simulink model "CarE_Model"  (R2019b)
settings: Solver=VariableStepAuto  StartTime=0.0  StopTime=inf  RelTol=1e-3
(part 2 of 5)

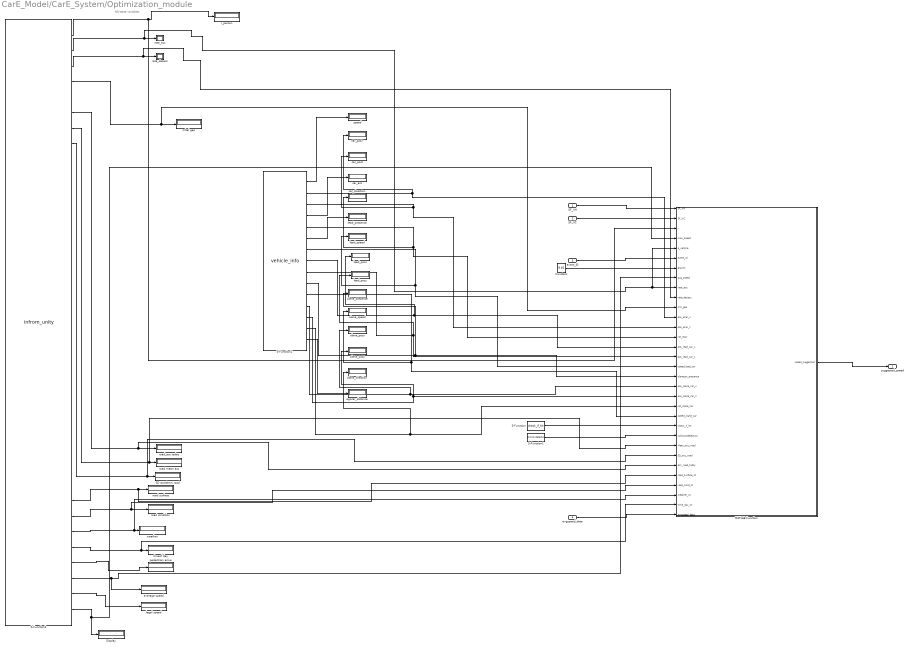
== system CarE_Model/CarE_System/Optimization_module ==
  note: NO-state variables
  SF_VH : Inport
  SF_VC : Inport  Port=2
  event_ID : Inport  Port=3
  avgspeed_data : Inport  Port=4
  Constant : Constant  Value=9.81
  Display : Display
  MATLAB Function : MATLAB Function  TreatAsAtomicUnit=on
  S-Function : S-Function  FunctionName=check_if_hit  SFunctionDeploymentMode=off  EnableBusSupport=off
  S-Function1 : S-Function  FunctionName=collisiondetection  SFunctionDeploymentMode=off  EnableBusSupport=off
  S-Function2 : S-Function  FunctionName=vehicle_info  SFunctionDeploymentMode=off  EnableBusSupport=off
  S-Function3 : S-Function  FunctionName=infrom_unity  SFunctionDeploymentMode=off  EnableBusSupport=off
  SD accidenrs road : Display
  average speed : Display
  car_acc : Display
  car_direction : Display
  car_posx : Display
  car_posz : Display
  crital gap : Display
  egocar_distance : Display
  lead_posx : Display
  lead_posz : Display
  lead_presence : Display
  lead_speed : Display
      settings: Decimation=5
  legal speed : Display
  olane_direction : Display
  olane_posx : Display
  olane_posz : Display
  olane_presence : Display
  olane_speed : Display
      settings: Decimation=5
  pedestrian acive : Display
  r_person : Display
  rate_acc : Display
  rate_desacc : Display
  road condition : Display
  road mean acc : Display
  road surface : Display
  road_acc today : Display
  speed : Display
      settings: Decimation=5
  timeof day : Display
  weather : Display
  suggested_speed : Outport
  wires:
  MATLAB Function/1(speed_suggestion) -> suggested_speed/1
  S-Function3/1 -> MATLAB Function/3(r), r_person/1
  SF_VC/1 -> MATLAB Function/2(SF_VC)
  SF_VH/1 -> MATLAB Function/1(SF_VH)
  S-Function3/38 -> MATLAB Function/4(max_speed), Display/1
  event_ID/1 -> MATLAB Function/6(event_id)
  Constant/1 -> MATLAB Function/7(gravity)
  S-Function3/36 -> average speed/1, MATLAB Function/8(avg_speed)
  S-Function3/2 -> MATLAB Function/5(a_vehicle), MATLAB Function/9(rate_acc), rate_acc/1
  S-Function3/3 -> MATLAB Function/10(rate_desacc), rate_desacc/1
  S-Function3/4 -> MATLAB Function/11(crit_gap), crital gap/1
  S-Function/1 -> MATLAB Function/23(check_if_hit)
  S-Function1/1 -> MATLAB Function/24(collisiondetection)
  S-Function3/7 -> MATLAB Function/25(Mean_acc_road), road mean acc/1
  S-Function3/8 -> MATLAB Function/26(SD_acc_road), SD accidenrs road/1
  S-Function3/6 -> MATLAB Function/27(acc_road_today), road_acc today/1
  S-Function3/31 -> MATLAB Function/28(road_surface_st), road surface/1
  S-Function3/32 -> MATLAB Function/29(road_cond_st), road condition/1
  S-Function3/33 -> MATLAB Function/30(weather_st), weather/1
  S-Function3/34 -> MATLAB Function/31(time_day_st), timeof day/1
  avgspeed_data/1 -> MATLAB Function/32(avgspeed_data)
  S-Function2/6 -> lead_presence/1
  S-Function2/11 -> MATLAB Function/22(speed_olane_car), olane_speed/1
  S-Function2/5 -> MATLAB Function/14(rot_ecar), car_direction/1
  S-Function2/8 -> MATLAB Function/15(pos_lead_car_x), lead_posx/1
  S-Function2/9 -> MATLAB Function/16(pos_lead_car_z), lead_posz/1
  S-Function2/12 -> MATLAB Function/19(pos_olane_car_x), olane_posx/1
  S-Function2/13 -> MATLAB Function/20(pos_olane_car_z), olane_posz/1
  S-Function2/15 -> egocar_distance/1
  S-Function2/7 -> MATLAB Function/17(speed_lead_car), lead_speed/1
  S-Function2/14 -> MATLAB Function/21(rot_olane_car), olane_direction/1
  S-Function2/2 -> MATLAB Function/12(pos_ecar_x), car_posx/1
  S-Function2/10 -> MATLAB Function/18(olanecar_presence), olane_presence/1
  S-Function2/3 -> MATLAB Function/13(pos_ecar_z), car_posz/1
  S-Function2/1 -> speed/1
  S-Function3/37 -> legal speed/1
  S-Function3/35 -> pedestrian acive/1
  S-Function2/4 -> car_acc/1

== system CarE_Model/CarE_System/Output Module ==
  mood : Inport
  anger_val : Inport  Port=2
  disgust_val : Inport  Port=3
  fear_val : Inport  Port=4
  happiness_val : Inport  Port=5
  neutral_val : Inport  Port=6
  sadness_val : Inport  Port=7
  surprise_val : Inport  Port=8
  stress_val : Inport  Port=9
  Body_mapping : Subsystem
  S-Function1 : S-Function  FunctionName=map_to_unity  SFunctionDeploymentMode=off  EnableBusSupport=off
  wires:
  mood/1 -> S-Function1/1
  anger_val/1 -> Body_mapping/1(anger), S-Function1/2
  disgust_val/1 -> Body_mapping/2(disgust), S-Function1/3
  fear_val/1 -> Body_mapping/3(fear), S-Function1/4
  happiness_val/1 -> Body_mapping/4(happiness), S-Function1/5
  neutral_val/1 -> Body_mapping/5(neutral), S-Function1/6
  sadness_val/1 -> Body_mapping/6(sadness), S-Function1/7
  surprise_val/1 -> Body_mapping/7(surprise), S-Function1/8
  stress_val/1 -> Body_mapping/8(stress), S-Function1/9

== system CarE_Model/CarE_System/Personality_module ==
  egocar_speed : Inport
  egocar_max_speed : Inport  Port=2
  r_personality : Inport  Port=3
  MATLAB Function : MATLAB Function  TreatAsAtomicUnit=on
  MATLAB Function1 : MATLAB Function  TreatAsAtomicUnit=on
  Utility : Outport
  wires:
  egocar_max_speed/1 -> MATLAB Function/2(max_speed)
  egocar_speed/1 -> MATLAB Function/1(speed)
  r_personality/1 -> MATLAB Function1/2(r)
  MATLAB Function/2(max_x) -> MATLAB Function1/3(max_x)
  MATLAB Function/1(x) -> MATLAB Function1/1(x)
  MATLAB Function1/1(U) -> Utility/1

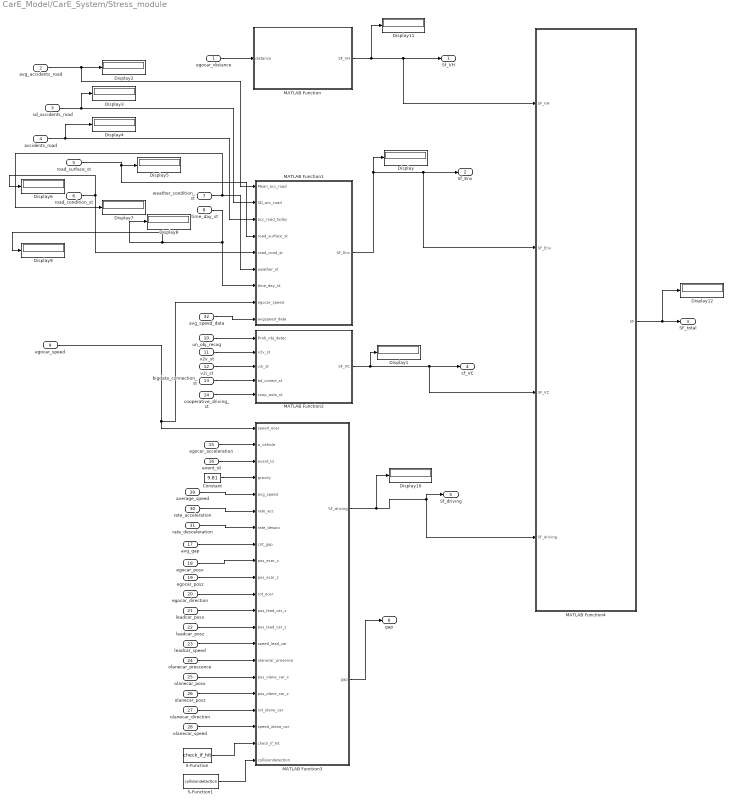
== system CarE_Model/CarE_System/Stress_module ==
  egocar_distance : Inport
  avg_accidents_road : Inport  Port=2
  sd_accidents_road : Inport  Port=3
  accidents_road : Inport  Port=4
  road_surface_st : Inport  Port=5
  road_condition_st : Inport  Port=6
  weather_condition_st : Inport  Port=7
  time_day_st : Inport  Port=8
  egocar_speed : Inport  Port=9
  un_obj_recog : Inport  Port=10
  v2v_st : Inport  Port=11
  v2i_st : Inport  Port=12
  bigdata_connection_st : Inport  Port=13
  cooperative_driving_st : Inport  Port=14
  egocar_acceleration : Inport  Port=15
  event_id : Inport  Port=16
  avg_gap : Inport  Port=17
  egocar_posx : Inport  Port=18
  egocar_posz : Inport  Port=19
  egocar_direction : Inport  Port=20
  leadcar_posx : Inport  Port=21
  leadcar_posz : Inport  Port=22
  leadcar_speed : Inport  Port=23
  olanecar_prescence : Inport  Port=24
  olanecar_posx : Inport  Port=25
  olanecar_posz : Inport  Port=26
  olanecar_direction : Inport  Port=27
  olanecar_speed : Inport  Port=28
  average_speed : Inport  Port=29
  rate_acceleration : Inport  Port=30
  rate_desceleration : Inport  Port=31
  avg_speed_data : Inport  Port=32
  Constant : Constant  Value=9.81
  Display{,1..12} (13 alike) : Display
  MATLAB Function : MATLAB Function  TreatAsAtomicUnit=on
  MATLAB Function1 : MATLAB Function  TreatAsAtomicUnit=on
  MATLAB Function2 : MATLAB Function  TreatAsAtomicUnit=on
  MATLAB Function3 : MATLAB Function  TreatAsAtomicUnit=on
  MATLAB Function4 : MATLAB Function  TreatAsAtomicUnit=on
  S-Function : S-Function  FunctionName=check_if_hit  SFunctionDeploymentMode=off  EnableBusSupport=off
  S-Function1 : S-Function  FunctionName=collisiondetection  SFunctionDeploymentMode=off  EnableBusSupport=off
  Sf_VH : Outport
  Sf_Env : Outport  Port=2
  SF_total : Outport  Port=3
  sf_VC : Outport  Port=4
  Sf_driving : Outport  Port=5
  gap : Outport  Port=6
  wires:
  MATLAB Function/1(SF_VH) -> Display11/1, MATLAB Function4/1(SF_VH), Sf_VH/1
  egocar_distance/1 -> MATLAB Function/1(distance)
  egocar_speed/1 -> MATLAB Function1/8(egocar_speed), MATLAB Function3/1(speed_ecar)
  avg_accidents_road/1 -> MATLAB Function1/1(Mean_acc_road), Display2/1
  sd_accidents_road/1 -> MATLAB Function1/2(SD_acc_road), Display3/1
  accidents_road/1 -> Display4/1, MATLAB Function1/3(acc_road_today)
  road_surface_st/1 -> MATLAB Function1/4(road_surface_st), Display5/1
  road_condition_st/1 -> Display6/1, MATLAB Function1/5(road_cond_st)
  weather_condition_st/1 -> Display7/1, MATLAB Function1/6(weather_st)
  time_day_st/1 -> Display9/1, Display8/1, MATLAB Function1/7(time_day_st)
  MATLAB Function1/1(SF_Env) -> Display/1, MATLAB Function4/2(SF_Env), Sf_Env/1
  MATLAB Function4/1(SF) -> Display12/1, SF_total/1
  MATLAB Function2/1(SF_VC) -> Display1/1, MATLAB Function4/3(SF_VC), sf_VC/1
  MATLAB Function3/1(SF_driving) -> Display10/1, Sf_driving/1, MATLAB Function4/4(SF_driving)
  cooperative_driving_st/1 -> MATLAB Function2/5(coop_auto_st)
  bigdata_connection_st/1 -> MATLAB Function2/4(bd_conect_st)
  v2i_st/1 -> MATLAB Function2/3(v2i_st)
  v2v_st/1 -> MATLAB Function2/2(v2v_st)
  un_obj_recog/1 -> MATLAB Function2/1(Prob_obj_detec)
  Constant/1 -> MATLAB Function3/4(gravity)
  event_id/1 -> MATLAB Function3/3(event_id)
  egocar_acceleration/1 -> MATLAB Function3/2(a_vehicle)
  avg_gap/1 -> MATLAB Function3/8(crit_gap)
  leadcar_speed/1 -> MATLAB Function3/14(speed_lead_car)
  leadcar_posz/1 -> MATLAB Function3/13(pos_lead_car_z)
  leadcar_posx/1 -> MATLAB Function3/12(pos_lead_car_x)
  egocar_direction/1 -> MATLAB Function3/11(rot_ecar)
  egocar_posz/1 -> MATLAB Function3/10(pos_ecar_z)
  egocar_posx/1 -> MATLAB Function3/9(pos_ecar_x)
  olanecar_speed/1 -> MATLAB Function3/19(speed_olane_car)
  olanecar_direction/1 -> MATLAB Function3/18(rot_olane_car)
  olanecar_posz/1 -> MATLAB Function3/17(pos_olane_car_z)
  olanecar_posx/1 -> MATLAB Function3/16(pos_olane_car_x)
  olanecar_prescence/1 -> MATLAB Function3/15(olanecar_presence)
  MATLAB Function3/2(gap) -> gap/1
  rate_desceleration/1 -> MATLAB Function3/7(rate_desacc)
  rate_acceleration/1 -> MATLAB Function3/6(rate_acc)
  average_speed/1 -> MATLAB Function3/5(avg_speed)
  S-Function/1 -> MATLAB Function3/20(check_if_hit)
  S-Function1/1 -> MATLAB Function3/21(collisiondetection)
  avg_speed_data/1 -> MATLAB Function1/9(avgspeed_data)

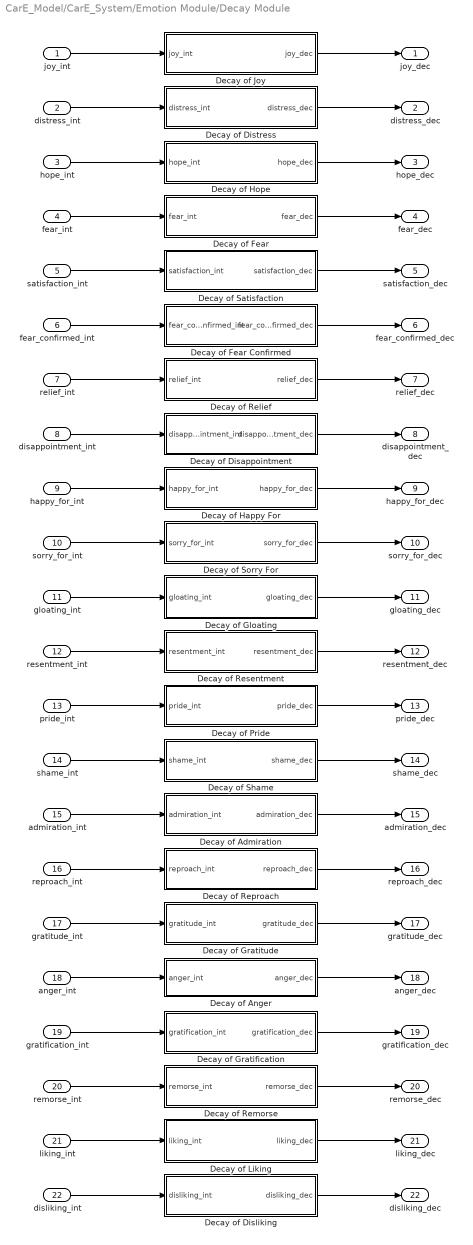
== system CarE_Model/CarE_System/Emotion Module/Decay Module ==
  joy_int : Inport
  distress_int : Inport  Port=2
  hope_int : Inport  Port=3
  fear_int : Inport  Port=4
  satisfaction_int : Inport  Port=5
  fear_confirmed_int : Inport  Port=6
  relief_int : Inport  Port=7
  disappointment_int : Inport  Port=8
  happy_for_int : Inport  Port=9
  sorry_for_int : Inport  Port=10
  gloating_int : Inport  Port=11
  resentment_int : Inport  Port=12
  pride_int : Inport  Port=13
  shame_int : Inport  Port=14
  admiration_int : Inport  Port=15
  reproach_int : Inport  Port=16
  gratitude_int : Inport  Port=17
  anger_int : Inport  Port=18
  gratification_int : Inport  Port=19
  remorse_int : Inport  Port=20
  liking_int : Inport  Port=21
  disliking_int : Inport  Port=22
  Decay of Admiration : Subsystem
  Decay of Anger : Subsystem
  Decay of Disappointment : Subsystem
  Decay of Disliking : Subsystem
  Decay of Distress : Subsystem
  Decay of Fear : Subsystem
  Decay of Fear Confirmed : Subsystem
  Decay of Gloating : Subsystem
  Decay of Gratification : Subsystem
  Decay of Gratitude : Subsystem
  Decay of Happy For : Subsystem
  Decay of Hope : Subsystem
  Decay of Joy : Subsystem
  Decay of Liking : Subsystem
  Decay of Pride : Subsystem
  Decay of Relief : Subsystem
  Decay of Remorse : Subsystem
  Decay of Reproach : Subsystem
  Decay of Resentment : Subsystem
  Decay of Satisfaction : Subsystem
  Decay of Shame : Subsystem
  Decay of Sorry For : Subsystem
  joy_dec : Outport  VectorParamsAs1DForOutWhenUnconnected=off
  "distress_dec " : Outport  Port=2  VectorParamsAs1DForOutWhenUnconnected=off
  hope_dec : Outport  Port=3  VectorParamsAs1DForOutWhenUnconnected=off
  fear_dec : Outport  Port=4  VectorParamsAs1DForOutWhenUnconnected=off
  satisfaction_dec : Outport  Port=5  VectorParamsAs1DForOutWhenUnconnected=off
  fear_confirmed_dec : Outport  Port=6  VectorParamsAs1DForOutWhenUnconnected=off
  relief_dec : Outport  Port=7  VectorParamsAs1DForOutWhenUnconnected=off
  disappointment_dec : Outport  Port=8  VectorParamsAs1DForOutWhenUnconnected=off
  happy_for_dec : Outport  Port=9  VectorParamsAs1DForOutWhenUnconnected=off
  sorry_for_dec : Outport  Port=10  VectorParamsAs1DForOutWhenUnconnected=off
  gloating_dec : Outport  Port=11  VectorParamsAs1DForOutWhenUnconnected=off
  resentment_dec : Outport  Port=12  VectorParamsAs1DForOutWhenUnconnected=off
  pride_dec : Outport  Port=13  VectorParamsAs1DForOutWhenUnconnected=off
  shame_dec : Outport  Port=14  VectorParamsAs1DForOutWhenUnconnected=off
  admiration_dec : Outport  Port=15  VectorParamsAs1DForOutWhenUnconnected=off
  reproach_dec : Outport  Port=16  VectorParamsAs1DForOutWhenUnconnected=off
  gratitude_dec : Outport  Port=17  VectorParamsAs1DForOutWhenUnconnected=off
  anger_dec : Outport  Port=18  VectorParamsAs1DForOutWhenUnconnected=off
  gratification_dec : Outport  Port=19  VectorParamsAs1DForOutWhenUnconnected=off
  remorse_dec : Outport  Port=20  VectorParamsAs1DForOutWhenUnconnected=off
  liking_dec : Outport  Port=21  VectorParamsAs1DForOutWhenUnconnected=off
  disliking_dec : Outport  Port=22  VectorParamsAs1DForOutWhenUnconnected=off
  wires:
  distress_int/1 -> Decay of Distress/1(distress_int)
  joy_int/1 -> Decay of Joy/1(joy_int)
  fear_int/1 -> Decay of Fear/1(fear_int)
  hope_int/1 -> Decay of Hope/1(hope_int)
  satisfaction_int/1 -> Decay of Satisfaction/1(satisfaction_int)
  fear_confirmed_int/1 -> Decay of Fear Confirmed/1(fear_confirmed_int)
  relief_int/1 -> Decay of Relief/1(relief_int)
  disappointment_int/1 -> Decay of Disappointment/1(disappointment_int)
  happy_for_int/1 -> Decay of Happy For/1(happy_for_int)
  sorry_for_int/1 -> Decay of Sorry For/1(sorry_for_int)
  gloating_int/1 -> Decay of Gloating/1(gloating_int)
  resentment_int/1 -> Decay of Resentment/1(resentment_int)
  pride_int/1 -> Decay of Pride/1(pride_int)
  shame_int/1 -> Decay of Shame/1(shame_int)
  admiration_int/1 -> Decay of Admiration/1(admiration_int)
  reproach_int/1 -> Decay of Reproach/1(reproach_int)
  gratitude_int/1 -> Decay of Gratitude/1(gratitude_int)
  anger_int/1 -> Decay of Anger/1(anger_int)
  gratification_int/1 -> Decay of Gratification/1(gratification_int)
  remorse_int/1 -> Decay of Remorse/1(remorse_int)
  liking_int/1 -> Decay of Liking/1(liking_int)
  disliking_int/1 -> Decay of Disliking/1(disliking_int)
  Decay of Joy/1(joy_dec) -> joy_dec/1
  Decay of Distress/1(distress_dec) -> "distress_dec "/1
  Decay of Hope/1(hope_dec) -> hope_dec/1
  Decay of Fear/1(fear_dec) -> fear_dec/1
  Decay of Satisfaction/1(satisfaction_dec) -> satisfaction_dec/1
  Decay of Fear Confirmed/1(fear_confirmed_dec) -> fear_confirmed_dec/1
  Decay of Relief/1(relief_dec) -> relief_dec/1
  Decay of Disappointment/1(disappointment_dec) -> disappointment_dec/1
  Decay of Happy For/1(happy_for_dec) -> happy_for_dec/1
  Decay of Sorry For/1(sorry_for_dec) -> sorry_for_dec/1
  Decay of Gloating/1(gloating_dec) -> gloating_dec/1
  Decay of Resentment/1(resentment_dec) -> resentment_dec/1
  Decay of Pride/1(pride_dec) -> pride_dec/1
  Decay of Shame/1(shame_dec) -> shame_dec/1
  Decay of Admiration/1(admiration_dec) -> admiration_dec/1
  Decay of Reproach/1(reproach_dec) -> reproach_dec/1
  Decay of Gratitude/1(gratitude_dec) -> gratitude_dec/1
  Decay of Anger/1(anger_dec) -> anger_dec/1
  Decay of Gratification/1(gratification_dec) -> gratification_dec/1
  Decay of Remorse/1(remorse_dec) -> remorse_dec/1
  Decay of Liking/1(liking_dec) -> liking_dec/1
  Decay of Disliking/1(disliking_dec) -> disliking_dec/1

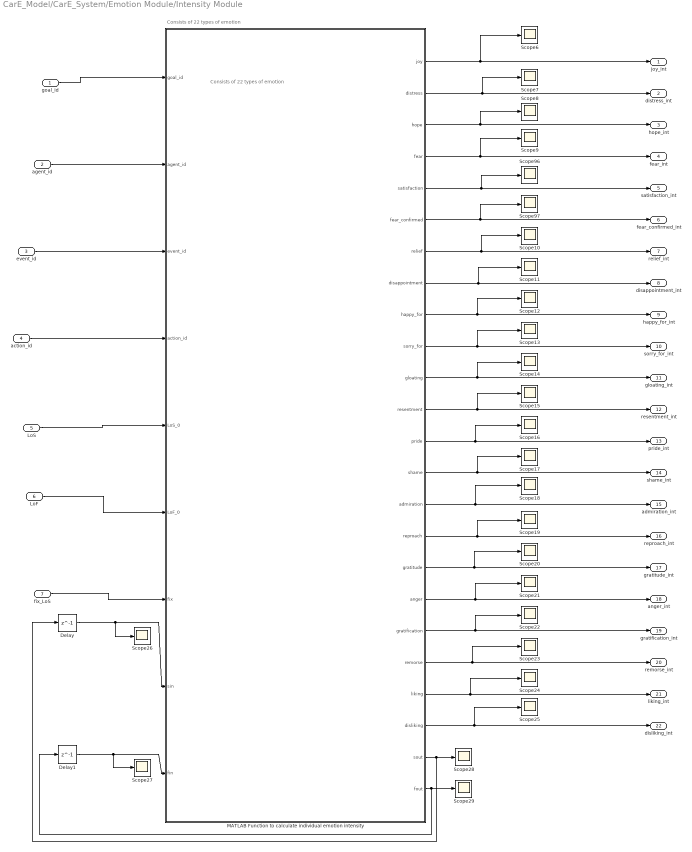
== system CarE_Model/CarE_System/Emotion Module/Intensity Module ==
  note: Consists of 22 types of emotion
  note: Consists of 22 types of emotion
  goal_id : Inport
  agent_id : Inport  Port=2
  event_id : Inport  Port=3
  action_id : Inport  Port=4
  LoS : Inport  Port=5
  LoF : Inport  Port=6
  fix_LoS : Inport  Port=7
  Delay : Delay  DelayLength=1  InitialCondition=0
  Delay1 : Delay  DelayLength=1  InitialCondition=0
  MATLAB Function to calculate individual emotion intensity : MATLAB Function  TreatAsAtomicUnit=on
  Scope{6..29,96..97} (26 alike) : Scope
  joy_int : Outport  VectorParamsAs1DForOutWhenUnconnected=off
  "distress_int " : Outport  Port=2  VectorParamsAs1DForOutWhenUnconnected=off
  hope_int : Outport  Port=3  VectorParamsAs1DForOutWhenUnconnected=off
  fear_int : Outport  Port=4  VectorParamsAs1DForOutWhenUnconnected=off
  satisfaction_int : Outport  Port=5  VectorParamsAs1DForOutWhenUnconnected=off
  fear_confirmed_int : Outport  Port=6  VectorParamsAs1DForOutWhenUnconnected=off
  relief_int : Outport  Port=7  VectorParamsAs1DForOutWhenUnconnected=off
  disappointment_int : Outport  Port=8  VectorParamsAs1DForOutWhenUnconnected=off
  happy_for_int : Outport  Port=9  VectorParamsAs1DForOutWhenUnconnected=off
  sorry_for_int : Outport  Port=10  VectorParamsAs1DForOutWhenUnconnected=off
  gloating_int : Outport  Port=11  VectorParamsAs1DForOutWhenUnconnected=off
  resentment_int : Outport  Port=12  VectorParamsAs1DForOutWhenUnconnected=off
  pride_int : Outport  Port=13  VectorParamsAs1DForOutWhenUnconnected=off
  shame_int : Outport  Port=14  VectorParamsAs1DForOutWhenUnconnected=off
  admiration_int : Outport  Port=15  VectorParamsAs1DForOutWhenUnconnected=off
  reproach_int : Outport  Port=16  VectorParamsAs1DForOutWhenUnconnected=off
  gratitude_int : Outport  Port=17  VectorParamsAs1DForOutWhenUnconnected=off
  anger_int : Outport  Port=18  VectorParamsAs1DForOutWhenUnconnected=off
  gratification_int : Outport  Port=19  VectorParamsAs1DForOutWhenUnconnected=off
  remorse_int : Outport  Port=20  VectorParamsAs1DForOutWhenUnconnected=off
  liking_int : Outport  Port=21  VectorParamsAs1DForOutWhenUnconnected=off
  disliking_int : Outport  Port=22  VectorParamsAs1DForOutWhenUnconnected=off
  wires:
  MATLAB Function to calculate individual emotion intensity/11(gloating) -> gloating_int/1, Scope14/1
  MATLAB Function to calculate individual emotion intensity/9(happy_for) -> happy_for_int/1, Scope12/1
  event_id/1 -> MATLAB Function to calculate individual emotion intensity/3(event_id)
  MATLAB Function to calculate individual emotion intensity/10(sorry_for) -> sorry_for_int/1, Scope13/1
  goal_id/1 -> MATLAB Function to calculate individual emotion intensity/1(goal_id)
  MATLAB Function to calculate individual emotion intensity/4(fear) -> fear_int/1, Scope9/1
  MATLAB Function to calculate individual emotion intensity/3(hope) -> hope_int/1, Scope8/1
  MATLAB Function to calculate individual emotion intensity/19(gratification) -> gratification_int/1, Scope22/1
  MATLAB Function to calculate individual emotion intensity/13(pride) -> pride_int/1, Scope16/1
  MATLAB Function to calculate individual emotion intensity/20(remorse) -> remorse_int/1, Scope23/1
  Delay/1 -> Scope26/1, MATLAB Function to calculate individual emotion intensity/8(sin)
  MATLAB Function to calculate individual emotion intensity/17(gratitude) -> gratitude_int/1, Scope20/1
  MATLAB Function to calculate individual emotion intensity/22(disliking) -> disliking_int/1, Scope25/1
  MATLAB Function to calculate individual emotion intensity/21(liking) -> Scope24/1, liking_int/1
  MATLAB Function to calculate individual emotion intensity/8(disappointment) -> disappointment_int/1, Scope11/1
  MATLAB Function to calculate individual emotion intensity/2(distress) -> "distress_int "/1, Scope7/1
  MATLAB Function to calculate individual emotion intensity/15(admiration) -> admiration_int/1, Scope18/1
  MATLAB Function to calculate individual emotion intensity/5(satisfaction) -> satisfaction_int/1, Scope96/1
  MATLAB Function to calculate individual emotion intensity/18(anger) -> anger_int/1, Scope21/1
  agent_id/1 -> MATLAB Function to calculate individual emotion intensity/2(agent_id)
  MATLAB Function to calculate individual emotion intensity/6(fear_confirmed) -> fear_confirmed_int/1, Scope97/1
  Delay1/1 -> Scope27/1, MATLAB Function to calculate individual emotion intensity/9(fin)
  MATLAB Function to calculate individual emotion intensity/1(joy) -> joy_int/1, Scope6/1
  MATLAB Function to calculate individual emotion intensity/16(reproach) -> reproach_int/1, Scope19/1
  action_id/1 -> MATLAB Function to calculate individual emotion intensity/4(action_id)
  MATLAB Function to calculate individual emotion intensity/12(resentment) -> resentment_int/1, Scope15/1
  MATLAB Function to calculate individual emotion intensity/14(shame) -> shame_int/1, Scope17/1
  MATLAB Function to calculate individual emotion intensity/24(fout) -> Delay1/1, Scope29/1
  MATLAB Function to calculate individual emotion intensity/7(relief) -> relief_int/1, Scope10/1
  MATLAB Function to calculate individual emotion intensity/23(sout) -> Delay/1, Scope28/1
  LoS/1 -> MATLAB Function to calculate individual emotion intensity/5(LoS_0)
  LoF/1 -> MATLAB Function to calculate individual emotion intensity/6(LoF_0)
  fix_LoS/1 -> MATLAB Function to calculate individual emotion intensity/7(fix)

== system CarE_Model/CarE_System/Output Module/Body_mapping ==
  anger : Inport
  disgust : Inport  Port=2
  fear : Inport  Port=3
  happiness : Inport  Port=4
  neutral : Inport  Port=5
  sadness : Inport  Port=6
  surprise : Inport  Port=7
  stress : Inport  Port=8
  MATLAB Function : MATLAB Function  TreatAsAtomicUnit=on
  S-Function : S-Function  FunctionName=bodymap  SFunctionDeploymentMode=off  EnableBusSupport=off
  wires:
  stress/1 -> MATLAB Function/8(stress)
  surprise/1 -> MATLAB Function/7(surprise)
  sadness/1 -> MATLAB Function/6(sadness)
  neutral/1 -> MATLAB Function/5(neutral)
  happiness/1 -> MATLAB Function/4(happiness)
  fear/1 -> MATLAB Function/3(fear)
  disgust/1 -> MATLAB Function/2(disgust)
  anger/1 -> MATLAB Function/1(anger)
  MATLAB Function/1(cabine_st) -> S-Function/1
  MATLAB Function/2(tires_st) -> S-Function/2
  MATLAB Function/3(wheels_st) -> S-Function/3
  MATLAB Function/4(motor_st) -> S-Function/4
  MATLAB Function/5(dashboard_st) -> S-Function/5
  MATLAB Function/6(door_st) -> S-Function/6
  MATLAB Function/7(body_st) -> S-Function/7
  MATLAB Function/8(windshield_st) -> S-Function/8
  MATLAB Function/9(ligths_st) -> S-Function/9
  MATLAB Function/10(comm_st) -> S-Function/10

== system CarE_Model/CarE_System/Emotion Module/Decay Module/Decay of Admiration ==
  admiration_int : Inport
  Clock : Clock
  Delay : Delay  DelayLength=1  InitialCondition=0
  MATLAB Function : MATLAB Function  TreatAsAtomicUnit=on
  admiration_dec : Outport  VectorParamsAs1DForOutWhenUnconnected=off
  wires:
  admiration_int/1 -> Delay/1, MATLAB Function/1(u)
  Clock/1 -> MATLAB Function/2(t)
  MATLAB Function/1(y) -> admiration_dec/1
  Delay/1 -> MATLAB Function/3(ulast)

== system CarE_Model/CarE_System/Emotion Module/Decay Module/Decay of Anger ==
  anger_int : Inport
  Clock : Clock
  Delay : Delay  DelayLength=1  InitialCondition=0
  MATLAB Function : MATLAB Function  TreatAsAtomicUnit=on
  anger_dec : Outport  VectorParamsAs1DForOutWhenUnconnected=off
  wires:
  Delay/1 -> MATLAB Function/3(ulast)
  Clock/1 -> MATLAB Function/2(t)
  anger_int/1 -> Delay/1, MATLAB Function/1(u)
  MATLAB Function/1(y) -> anger_dec/1

== system CarE_Model/CarE_System/Emotion Module/Decay Module/Decay of Disappointment ==
  disappointment_int : Inport
  Clock : Clock
  Delay : Delay  DelayLength=1  InitialCondition=0
  MATLAB Function : MATLAB Function  TreatAsAtomicUnit=on
  disappointment_dec : Outport  VectorParamsAs1DForOutWhenUnconnected=off
  wires:
  Delay/1 -> MATLAB Function/3(ulast)
  Clock/1 -> MATLAB Function/2(t)
  disappointment_int/1 -> Delay/1, MATLAB Function/1(u)
  MATLAB Function/1(y) -> disappointment_dec/1

== system CarE_Model/CarE_System/Emotion Module/Decay Module/Decay of Disliking ==
  disliking_int : Inport
  Clock : Clock
  Delay : Delay  DelayLength=1  InitialCondition=0
  MATLAB Function : MATLAB Function  TreatAsAtomicUnit=on
  disliking_dec : Outport  VectorParamsAs1DForOutWhenUnconnected=off
  wires:
  Delay/1 -> MATLAB Function/3(ulast)
  Clock/1 -> MATLAB Function/2(t)
  disliking_int/1 -> Delay/1, MATLAB Function/1(u)
  MATLAB Function/1(y) -> disliking_dec/1

== system CarE_Model/CarE_System/Emotion Module/Decay Module/Decay of Distress ==
  distress_int : Inport
  Clock : Clock
  Delay : Delay  DelayLength=1  InitialCondition=0
  MATLAB Function : MATLAB Function  TreatAsAtomicUnit=on
  distress_dec : Outport  VectorParamsAs1DForOutWhenUnconnected=off
  wires:
  Clock/1 -> MATLAB Function/2(t)
  MATLAB Function/1(y) -> distress_dec/1
  Delay/1 -> MATLAB Function/3(ulast)
  distress_int/1 -> Delay/1, MATLAB Function/1(u)

== system CarE_Model/CarE_System/Emotion Module/Decay Module/Decay of Fear ==
  fear_int : Inport
  Clock : Clock
  Delay : Delay  DelayLength=1  InitialCondition=0
  MATLAB Function : MATLAB Function  TreatAsAtomicUnit=on
  fear_dec : Outport  VectorParamsAs1DForOutWhenUnconnected=off
  wires:
  Delay/1 -> MATLAB Function/3(ulast)
  Clock/1 -> MATLAB Function/2(t)
  fear_int/1 -> Delay/1, MATLAB Function/1(u)
  MATLAB Function/1(y) -> fear_dec/1

== system CarE_Model/CarE_System/Emotion Module/Decay Module/Decay of Fear Confirmed ==
  fear_confirmed_int : Inport
  Clock : Clock
  Delay : Delay  DelayLength=1  InitialCondition=0
  MATLAB Function : MATLAB Function  TreatAsAtomicUnit=on
  fear_confirmed_dec : Outport  VectorParamsAs1DForOutWhenUnconnected=off
  wires:
  Delay/1 -> MATLAB Function/3(ulast)
  Clock/1 -> MATLAB Function/2(t)
  fear_confirmed_int/1 -> Delay/1, MATLAB Function/1(u)
  MATLAB Function/1(y) -> fear_confirmed_dec/1

== system CarE_Model/CarE_System/Emotion Module/Decay Module/Decay of Gloating ==
  gloating_int : Inport
  Clock : Clock
  Delay : Delay  DelayLength=1  InitialCondition=0
  MATLAB Function : MATLAB Function  TreatAsAtomicUnit=on
  gloating_dec : Outport  VectorParamsAs1DForOutWhenUnconnected=off
  wires:
  Delay/1 -> MATLAB Function/3(ulast)
  Clock/1 -> MATLAB Function/2(t)
  gloating_int/1 -> Delay/1, MATLAB Function/1(u)
  MATLAB Function/1(y) -> gloating_dec/1

== system CarE_Model/CarE_System/Emotion Module/Decay Module/Decay of Gratification ==
  gratification_int : Inport
  Clock : Clock
  Delay : Delay  DelayLength=1  InitialCondition=0
  MATLAB Function : MATLAB Function  TreatAsAtomicUnit=on
  gratification_dec : Outport  VectorParamsAs1DForOutWhenUnconnected=off
  wires:
  Delay/1 -> MATLAB Function/3(ulast)
  Clock/1 -> MATLAB Function/2(t)
  gratification_int/1 -> Delay/1, MATLAB Function/1(u)
  MATLAB Function/1(y) -> gratification_dec/1

== system CarE_Model/CarE_System/Emotion Module/Decay Module/Decay of Gratitude ==
  gratitude_int : Inport
  Clock : Clock
  Delay : Delay  DelayLength=1  InitialCondition=0
  MATLAB Function : MATLAB Function  TreatAsAtomicUnit=on
  gratitude_dec : Outport  VectorParamsAs1DForOutWhenUnconnected=off
  wires:
  Delay/1 -> MATLAB Function/3(ulast)
  Clock/1 -> MATLAB Function/2(t)
  gratitude_int/1 -> Delay/1, MATLAB Function/1(u)
  MATLAB Function/1(y) -> gratitude_dec/1

== system CarE_Model/CarE_System/Emotion Module/Decay Module/Decay of Happy For ==
  happy_for_int : Inport
  Clock : Clock
  Delay : Delay  DelayLength=1  InitialCondition=0
  MATLAB Function : MATLAB Function  TreatAsAtomicUnit=on
  happy_for_dec : Outport  VectorParamsAs1DForOutWhenUnconnected=off
  wires:
  Delay/1 -> MATLAB Function/3(ulast)
  Clock/1 -> MATLAB Function/2(t)
  happy_for_int/1 -> Delay/1, MATLAB Function/1(u)
  MATLAB Function/1(y) -> happy_for_dec/1

== system CarE_Model/CarE_System/Emotion Module/Decay Module/Decay of Hope ==
  hope_int : Inport
  Clock : Clock
  Delay : Delay  DelayLength=1  InitialCondition=0
  MATLAB Function : MATLAB Function  TreatAsAtomicUnit=on
  hope_dec : Outport  VectorParamsAs1DForOutWhenUnconnected=off
  wires:
  Delay/1 -> MATLAB Function/3(ulast)
  Clock/1 -> MATLAB Function/2(t)
  hope_int/1 -> Delay/1, MATLAB Function/1(u)
  MATLAB Function/1(y) -> hope_dec/1

== system CarE_Model/CarE_System/Emotion Module/Decay Module/Decay of Joy ==
  note: after every new value of emotion, the time must reset to zero
  joy_int : Inport
  Clock1 : Clock
  Delay : Delay  DelayLength=1  InitialCondition=0
  MATLAB Function1 : MATLAB Function  TreatAsAtomicUnit=on
  joy_dec : Outport  VectorParamsAs1DForOutWhenUnconnected=off
  wires:
  Clock1/1 -> MATLAB Function1/2(t)
  MATLAB Function1/1(y) -> joy_dec/1
  Delay/1 -> MATLAB Function1/3(ulast)
  joy_int/1 -> Delay/1, MATLAB Function1/1(u)

== system CarE_Model/CarE_System/Emotion Module/Decay Module/Decay of Liking ==
  liking_int : Inport
  Clock : Clock
  Delay : Delay  DelayLength=1  InitialCondition=0
  MATLAB Function : MATLAB Function  TreatAsAtomicUnit=on
  liking_dec : Outport  VectorParamsAs1DForOutWhenUnconnected=off
  wires:
  Delay/1 -> MATLAB Function/3(ulast)
  Clock/1 -> MATLAB Function/2(t)
  liking_int/1 -> Delay/1, MATLAB Function/1(u)
  MATLAB Function/1(y) -> liking_dec/1

== system CarE_Model/CarE_System/Emotion Module/Decay Module/Decay of Pride ==
  pride_int : Inport
  Clock : Clock
  Delay : Delay  DelayLength=1  InitialCondition=0
  MATLAB Function : MATLAB Function  TreatAsAtomicUnit=on
  pride_dec : Outport  VectorParamsAs1DForOutWhenUnconnected=off
  wires:
  Delay/1 -> MATLAB Function/3(ulast)
  Clock/1 -> MATLAB Function/2(t)
  pride_int/1 -> Delay/1, MATLAB Function/1(u)
  MATLAB Function/1(y) -> pride_dec/1

== system CarE_Model/CarE_System/Emotion Module/Decay Module/Decay of Relief ==
  relief_int : Inport
  Clock : Clock
  Delay : Delay  DelayLength=1  InitialCondition=0
  MATLAB Function : MATLAB Function  TreatAsAtomicUnit=on
  relief_dec : Outport  VectorParamsAs1DForOutWhenUnconnected=off
  wires:
  Delay/1 -> MATLAB Function/3(ulast)
  Clock/1 -> MATLAB Function/2(t)
  relief_int/1 -> Delay/1, MATLAB Function/1(u)
  MATLAB Function/1(y) -> relief_dec/1

== system CarE_Model/CarE_System/Emotion Module/Decay Module/Decay of Remorse ==
  remorse_int : Inport
  Clock : Clock
  Delay : Delay  DelayLength=1  InitialCondition=0
  MATLAB Function : MATLAB Function  TreatAsAtomicUnit=on
  remorse_dec : Outport  VectorParamsAs1DForOutWhenUnconnected=off
  wires:
  Delay/1 -> MATLAB Function/3(ulast)
  Clock/1 -> MATLAB Function/2(t)
  remorse_int/1 -> Delay/1, MATLAB Function/1(u)
  MATLAB Function/1(y) -> remorse_dec/1

== system CarE_Model/CarE_System/Emotion Module/Decay Module/Decay of Reproach ==
  reproach_int : Inport
  Clock : Clock
  Delay : Delay  DelayLength=1  InitialCondition=0
  MATLAB Function : MATLAB Function  TreatAsAtomicUnit=on
  reproach_dec : Outport  VectorParamsAs1DForOutWhenUnconnected=off
  wires:
  Delay/1 -> MATLAB Function/3(ulast)
  Clock/1 -> MATLAB Function/2(t)
  reproach_int/1 -> Delay/1, MATLAB Function/1(u)
  MATLAB Function/1(y) -> reproach_dec/1

== system CarE_Model/CarE_System/Emotion Module/Decay Module/Decay of Resentment ==
  resentment_int : Inport
  Clock : Clock
  Delay : Delay  DelayLength=1  InitialCondition=0
  MATLAB Function : MATLAB Function  TreatAsAtomicUnit=on
  resentment_dec : Outport  VectorParamsAs1DForOutWhenUnconnected=off
  wires:
  Delay/1 -> MATLAB Function/3(ulast)
  Clock/1 -> MATLAB Function/2(t)
  resentment_int/1 -> Delay/1, MATLAB Function/1(u)
  MATLAB Function/1(y) -> resentment_dec/1

== system CarE_Model/CarE_System/Emotion Module/Decay Module/Decay of Satisfaction ==
  satisfaction_int : Inport
  Clock : Clock
  Delay : Delay  DelayLength=1  InitialCondition=0
  MATLAB Function : MATLAB Function  TreatAsAtomicUnit=on
  satisfaction_dec : Outport  VectorParamsAs1DForOutWhenUnconnected=off
  wires:
  Delay/1 -> MATLAB Function/3(ulast)
  Clock/1 -> MATLAB Function/2(t)
  satisfaction_int/1 -> Delay/1, MATLAB Function/1(u)
  MATLAB Function/1(y) -> satisfaction_dec/1

== system CarE_Model/CarE_System/Emotion Module/Decay Module/Decay of Shame ==
  shame_int : Inport
  Clock : Clock
  Delay : Delay  DelayLength=1  InitialCondition=0
  MATLAB Function : MATLAB Function  TreatAsAtomicUnit=on
  shame_dec : Outport  VectorParamsAs1DForOutWhenUnconnected=off
  wires:
  Delay/1 -> MATLAB Function/3(ulast)
  Clock/1 -> MATLAB Function/2(t)
  shame_int/1 -> Delay/1, MATLAB Function/1(u)
  MATLAB Function/1(y) -> shame_dec/1

== system CarE_Model/CarE_System/Emotion Module/Decay Module/Decay of Sorry For ==
  sorry_for_int : Inport
  Clock : Clock
  Delay : Delay  DelayLength=1  InitialCondition=0
  MATLAB Function : MATLAB Function  TreatAsAtomicUnit=on
  sorry_for_dec : Outport  VectorParamsAs1DForOutWhenUnconnected=off
  wires:
  Delay/1 -> MATLAB Function/3(ulast)
  Clock/1 -> MATLAB Function/2(t)
  sorry_for_int/1 -> Delay/1, MATLAB Function/1(u)
  MATLAB Function/1(y) -> sorry_for_dec/1
